simulink model "snb_b_ser2par"  (R2012b)
settings: Solver=FixedStepDiscrete  SolverMode=SingleTasking  StartTime=0.0  StopTime=10000  RelTol=1e-3
undefined symbols (not defined in the file): Down, pfb_coeff_gen_calc, Up, xlipgetpartsetting
libraries: xbsIndex_r4 x8784, casper_library_misc x9, casper_library_communications x8, casper_library_delays x1, xps_library x1
(part 19 of 57)

== system snb_b_ser2par/unpack_and_reorder/fifo1 ==
  note: We are done transmitting if
      | we have reached the end
      | of the data, or are in reset
  note: We start off in reset and hold
      | reset high till the end of the first
      | packet we receive
  note: we do not allow writes to the data buffer if we know
      | that we are going to discard the current packet
  note: The flag buffer stores the word count
      | and flag associated with each packet
      | received. This is used to extract the
      | correct number of words and tag
      | it appropriately on the way out
  note: a fifo overflow should never happen
      | as extra packets are discarded
      | and packets that are too large
      | are also discarded.
      | Kept as a a sanity check
  note: discard new packet
      | if packet count
      | indicates already
      | at max we can
      | store
  note: We have received a good packet if
      | 1. discard line is low for whole time
      | 2. eof is high
      | 3. rx word count is the expected
      | multiple
      | 4.  rx word count is less than the
      | maximum allowed
      | 5. not discarding current packet due
      | to packet limit reached
      | 6. en is high
  note: clear discard on
      | last word of packet
  note: count up on last item of packet,
      | count down as last word leaves,
      | leave as is if both
  note: change tlag
      | as last data
      |  word leaves
  rst : Inport
  din : Inport  Port=2
  eof : Inport  Port=3
  en : Inport  Port=4
  discard : Inport  Port=5
  flagi : Inport  Port=6
  tx : Inport  Port=7
  Constant : xbsIndex_r4/Constant  const=2^scale_factor_bits-1  gui_display_data_type=Fixed-point  arith_type=Unsigned  n_bits=scale_factor_bits  bin_pt=0  preci_type=Single  exp_width=8  frac_width=24  explicit_period=on  period=1  equ=P=C  opselect=C  inp2=PCIN>>17  opr=+  inp1=P  carry=CIN  dbl_ovrd=off  block_type=constant
  Constant1 : xbsIndex_r4/Constant  const=0  gui_display_data_type=Boolean  arith_type=Boolean  n_bits=scale_factor_bits  bin_pt=0  preci_type=Single  exp_width=8  frac_width=24  explicit_period=on  period=1  equ=P=C  opselect=C  inp2=PCIN>>17  opr=+  inp1=P  carry=CIN  dbl_ovrd=off  block_type=constant
  Delay{,1..5,7..14} (14 alike) : xbsIndex_r4/Delay  rst=off  infoeditControl=Selection of Reset will increase slice count due to use of real FFs and instead of SRLs  en=off  latency=1  dbl_ovrd=off  reg_retiming=on  block_type=delay
      settings: block_version=11.4
  Delay6 : xbsIndex_r4/Delay  rst=on  infoeditControl=Selection of Reset will increase slice count due to use of real FFs and instead of SRLs  en=on  latency=1  dbl_ovrd=off  reg_retiming=on  block_type=delay
  Gateway Out{,1..20} (21 alike) : xbsIndex_r4/Gateway Out  inherit_from_input=off  hdl_port=on  timing_constraint=None  locs_specified=off  LOCs={}  UseAsDAC=off  DACChannel='1'  block_type=gatewayout
  Inverter{1..6} (6 alike) : xbsIndex_r4/Inverter  en=off  latency=0  dbl_ovrd=off  block_type=inv
  Logical{,3,5,11} (4 alike) : xbsIndex_r4/Logical  logical_function=AND  inputs=2  en=off  latency=0  precision=Full  arith_type=Unsigned  n_bits=16  bin_pt=0  align_bp=on  dbl_ovrd=off  block_type=logical
      Logical11 settings: block_version=11.4
  Logical1 : xbsIndex_r4/Logical  logical_function=AND  inputs=3  en=off  latency=0  precision=Full  arith_type=Unsigned  n_bits=16  bin_pt=0  align_bp=on  dbl_ovrd=off  block_type=logical
  Logical2 : xbsIndex_r4/Logical  logical_function=AND  inputs=6  en=off  latency=1  precision=Full  arith_type=Unsigned  n_bits=16  bin_pt=0  align_bp=on  dbl_ovrd=off  block_type=logical
  Logical{4,7..9} (4 alike) : xbsIndex_r4/Logical  logical_function=OR  inputs=2  en=off  latency=0  precision=Full  arith_type=Unsigned  n_bits=16  bin_pt=0  align_bp=on  dbl_ovrd=off  block_type=logical
      Logical7 settings: block_version=11.4
      Logical8 settings: block_version=11.4
      Logical9 settings: block_version=11.4
  Logical6 : xbsIndex_r4/Logical  logical_function=XOR  inputs=2  en=off  latency=0  precision=Full  arith_type=Unsigned  n_bits=16  bin_pt=0  align_bp=on  dbl_ovrd=off  block_type=logical
      settings: block_version=11.4
  Relational : xbsIndex_r4/Relational  mode=a=b  en=off  latency=0  dbl_ovrd=off  block_type=relational
  Slice : xbsIndex_r4/Slice  nbits=input_word_count_bits - scale_factor_bits  boolean_output=off  mode=Upper Bit Location + Width  bit1=0  base1=MSB of Input  bit0=0  base0=LSB of Input  dbl_ovrd=off  block_type=slice
  Terminator : Terminator
  Terminator1 : Terminator
  concat1 : xbsIndex_r4/Concat  num_inputs=2  dbl_ovrd=off  block_type=concat
  data_buffer : Subsystem  mask{depth_bits=input_word_count_bits+n_bits_depth, scale_factor=2^scale_factor_bits, full_bits=1, n_bits_in=n_bits_din, bram_latency=bram_latency}
      mask prompts: depth_bits "depth (2^?)"; scale_factor "output width scale factor"; full_bits "number of bits in %full signal"; n_bits_in "word size (bits)"; bram_latency "BRAM latency"
  discard_reg : xbsIndex_r4/Register  init=0  rst=on  en=on  dbl_ovrd=off  block_type=register
  discarding : xbsIndex_r4/Delay  rst=on  infoeditControl=Selection of Reset will increase slice count due to use of real FFs and instead of SRLs  en=on  latency=1  dbl_ovrd=off  reg_retiming=on  block_type=delay
      settings: block_version=11.4
  edge_detect : Subsystem  AncestorBlock=casper_library_misc/edge_detect  mask(edge_detect){edge=Rising, polarity=Active High, x_in=[0 0.08 0.08 0.16 0.16 0.24 0.24 0.32 0.32 0.4], y_in=[-1 -1  1  1  1  1  1  1  1  1], x_out=[0.6 0.68 0.68 0.76 0.76 0.84 0.84 0.92 0.92 1], y_out=[-1 -1  1  1 -1 -1 -1 -1 -1 -1]}
      mask prompts: edge "Edge Type"; polarity "Output Polarity"; x_in "Input X Positions"; y_in "Input Y Positions"; x_out "Output X Positions"; y_out "Output Y Positions"
      mask help: Output is active for one-cycle after each edge of the specified type (i.e. rising, falling or both).
      mask init: same as snb_b_ser2par/edge_detect
      settings: AttributesFormatString=|
      | rising edges
      | active high
      mask Help: Output is active for one-cycle after each edge of the specified type (i.e. rising, falling, or both).  Latency is zero.
      mask TypeOptions edge: Rising | Falling | Both
      mask TypeOptions polarity: Active High | Active Low
      mask Display:
      | plot(x_in_num,0.5+y_in_num*0.2);
      | plot(x_out_num,0.5+y_out_num*0.2);
  edge_detect1 : Subsystem  AncestorBlock=casper_library_misc/edge_detect  mask(edge_detect){edge=Falling, polarity=Active High, x_in=[0 0.08 0.08 0.16 0.16 0.24 0.24 0.32 0.32 0.4], y_in=[-1 -1  1  1  1  1  1  1  1  1], x_out=[0.6 0.68 0.68 0.76 0.76 0.84 0.84 0.92 0.92 1], y_out=[-1 -1  1  1 -1 -1 -1 -1 -1 -1]}
      mask prompts: edge "Edge Type"; polarity "Output Polarity"; x_in "Input X Positions"; y_in "Input Y Positions"; x_out "Output X Positions"; y_out "Output Y Positions"
      mask help: Output is active for one-cycle after each edge of the specified type (i.e. rising, falling or both).
      mask init: same as snb_b_ser2par/edge_detect
      settings: AttributesFormatString=|
      | falling edges
      | active high
      mask Help: Output is active for one-cycle after each edge of the specified type (i.e. rising, falling, or both).  Latency is zero.
      mask TypeOptions edge: Rising | Falling | Both
      mask TypeOptions polarity: Active High | Active Low
      mask Display:
      | plot(x_in_num,0.5+y_in_num*0.2);
      | plot(x_out_num,0.5+y_out_num*0.2);
  edge_detect2 : Subsystem  AncestorBlock=casper_library_misc/edge_detect  mask(edge_detect){edge=Rising, polarity=Active High, x_in=[0 0.08 0.08 0.16 0.16 0.24 0.24 0.32 0.32 0.4], y_in=[-1 -1  1  1  1  1  1  1  1  1], x_out=[0.6 0.68 0.68 0.76 0.76 0.84 0.84 0.92 0.92 1], y_out=[-1 -1  1  1 -1 -1 -1 -1 -1 -1]}
      mask prompts: edge "Edge Type"; polarity "Output Polarity"; x_in "Input X Positions"; y_in "Input Y Positions"; x_out "Output X Positions"; y_out "Output Y Positions"
      mask help: Output is active for one-cycle after each edge of the specified type (i.e. rising, falling or both).
      mask init: same as snb_b_ser2par/edge_detect
      settings: AttributesFormatString=|
      | rising edges
      | active high
      mask Help: Output is active for one-cycle after each edge of the specified type (i.e. rising, falling, or both).  Latency is zero.
      mask TypeOptions edge: Rising | Falling | Both
      mask TypeOptions polarity: Active High | Active Low
      mask Display:
      | plot(x_in_num,0.5+y_in_num*0.2);
      | plot(x_out_num,0.5+y_out_num*0.2);
  flag : xbsIndex_r4/Slice  nbits=n_bits_flag  boolean_output=off  mode=Lower Bit Location + Width  bit1=0  base1=MSB of Input  bit0=0  base0=LSB of Input  dbl_ovrd=off  block_type=slice
  flag_buffer : xbsIndex_r4/Dual Port RAM  depth=2^n_bits_depth  initVector=zeros(1, 2^n_bits_depth)  distributed_mem=Distributed memory  init_a=0  init_b=0  rst_a=off  rst_b=off  en_a=off  en_b=off  latency=1  write_mode_A=Read After Write  write_mode_B=Read After Write  dbl_ovrd=off  optimize=Area  block_type=dpram
  input : Scope  NumInputPorts=9
      settings: YMin=0~0~-1~0~3.25836e+46~5e+45~0~0~-5  YMax=1.2e+22~1~1~1~3.60134e+46~1.2e+46~1~750~5  SaveName=ScopeData4
  logical1 : xbsIndex_r4/Relational  mode=a=b  en=off  latency=0  dbl_ovrd=off  block_type=relational
  logical2 : xbsIndex_r4/Relational  mode=a>b  en=off  latency=1  dbl_ovrd=off  block_type=relational
  logical3 : xbsIndex_r4/Relational  mode=a=b  en=off  latency=1  dbl_ovrd=off  block_type=relational
  lsbs_wc : xbsIndex_r4/Slice  nbits=scale_factor_bits  boolean_output=off  mode=Lower Bit Location + Width  bit1=0  base1=MSB of Input  bit0=0  base0=LSB of Input  dbl_ovrd=off  block_type=slice
  msb_wc : xbsIndex_r4/Slice  nbits=1  boolean_output=on  mode=Upper Bit Location + Width  bit1=0  base1=MSB of Input  bit0=0  base0=LSB of Input  dbl_ovrd=off  block_type=slice
  output : Scope  NumInputPorts=7
      settings: YMin=-1~-1~-1~-1~-1~-1~-5  YMax=1~1~1~1~1~1~5  SaveName=ScopeData5
  output1 : Scope  NumInputPorts=5
      settings: YMin=0~0~0~0~0  YMax=1~1~600~1~300  SaveName=ScopeData8
  packet_count : xbsIndex_r4/Counter  cnt_type=Free Running  cnt_to=Inf  operation=Up/Down  start_count=0  cnt_by_val=1  arith_type=Unsigned  n_bits=n_bits_depth  bin_pt=0  load_pin=off  rst=on  en=on  explicit_period=on  period=1  dbl_ovrd=off  use_behavioral_HDL=on  implementation=Fabric  block_type=counter
  rd_add : xbsIndex_r4/Counter  cnt_type=Free Running  cnt_to=Inf  operation=Up  start_count=0  cnt_by_val=1  arith_type=Unsigned  n_bits=n_bits_depth  bin_pt=0  load_pin=off  rst=on  en=on  explicit_period=on  period=1  dbl_ovrd=off  use_behavioral_HDL=on  implementation=Fabric  block_type=counter
      settings: block_version=11.4
  rst_reg : xbsIndex_r4/Register  init=1  rst=on  en=on  dbl_ovrd=off  block_type=register
  word_count : xbsIndex_r4/Slice  nbits=input_word_count_bits  boolean_output=off  mode=Upper Bit Location + Width  bit1=0  base1=MSB of Input  bit0=0  base0=LSB of Input  dbl_ovrd=off  block_type=slice
  word_count1 : xbsIndex_r4/Slice  nbits=input_word_count_bits  boolean_output=off  mode=Lower Bit Location + Width  bit1=0  base1=MSB of Input  bit0=0  base0=LSB of Input  dbl_ovrd=off  block_type=slice
  word_count_in : xbsIndex_r4/Counter  cnt_type=Free Running  cnt_to=inf  operation=Up  start_count=0  cnt_by_val=1  arith_type=Unsigned  n_bits=input_word_count_bits + 1  bin_pt=0  load_pin=off  rst=on  en=on  explicit_period=on  period=1  dbl_ovrd=off  use_behavioral_HDL=on  implementation=Fabric  block_type=counter
  word_count_out : xbsIndex_r4/Counter  cnt_type=Free Running  cnt_to=inf  operation=Up  start_count=0  cnt_by_val=1  arith_type=Unsigned  n_bits=input_word_count_bits - scale_factor_bits  bin_pt=0  load_pin=off  rst=on  en=on  explicit_period=on  period=1  dbl_ovrd=off  use_behavioral_HDL=on  implementation=Fabric  block_type=counter
  wr_addr : xbsIndex_r4/Counter  cnt_type=Free Running  cnt_to=Inf  operation=Up  start_count=0  cnt_by_val=1  arith_type=Unsigned  n_bits=n_bits_depth  bin_pt=0  load_pin=off  rst=on  en=on  explicit_period=on  period=1  dbl_ovrd=off  use_behavioral_HDL=on  implementation=Fabric  block_type=counter
      settings: block_version=11.4
  zero : xbsIndex_r4/Constant  const=0  gui_display_data_type=Fixed-point  arith_type=Unsigned  n_bits=n_bits_depth  bin_pt=0  preci_type=Single  exp_width=8  frac_width=24  explicit_period=on  period=1  equ=P=C  opselect=C  inp2=PCIN>>17  opr=+  inp1=P  carry=CIN  dbl_ovrd=off  block_type=constant
  zero1 : xbsIndex_r4/Constant  const=0  gui_display_data_type=Fixed-point  arith_type=Unsigned  n_bits=2  bin_pt=0  preci_type=Single  exp_width=8  frac_width=24  explicit_period=on  period=1  equ=P=C  opselect=C  inp2=PCIN>>17  opr=+  inp1=P  carry=CIN  dbl_ovrd=off  block_type=constant
  zero2 : xbsIndex_r4/Constant  const=0  gui_display_data_type=Fixed-point  arith_type=Unsigned  n_bits=2  bin_pt=0  preci_type=Single  exp_width=8  frac_width=24  explicit_period=on  period=1  equ=P=C  opselect=C  inp2=PCIN>>17  opr=+  inp1=P  carry=CIN  dbl_ovrd=off  block_type=constant
  zero3 : xbsIndex_r4/Constant  const=2^n_bits_depth-1  gui_display_data_type=Fixed-point  arith_type=Unsigned  n_bits=n_bits_depth  bin_pt=0  preci_type=Single  exp_width=8  frac_width=24  explicit_period=on  period=1  equ=P=C  opselect=C  inp2=PCIN>>17  opr=+  inp1=P  carry=CIN  dbl_ovrd=off  block_type=constant
  dout : Outport
  flago : Outport  Port=2
  dvalid : Outport  Port=3
  done : Outport  Port=4
  ready : Outport  Port=5
  fifo_of : Outport  Port=6
  discading : Outport  Port=7
  wires:
  Logical/1 -> Logical8/2, discard_reg/3, discard_reg/1
  [rst_in] -> rd_add/1
  data_buffer/4(dvalid) -> Delay4/1, edge_detect1/1(in)
  wr_addr/1 -> Gateway Out3/1, flag_buffer/1
  en/1 -> Logical2/6, Delay14/1, word_count_in/2, Logical3/2, Logical/1, Delay2/1
  [rst_in] -> data_buffer/1(rst_rx)
  din/1 -> Delay1/1
  [rst_in] -> wr_addr/1
  data_buffer/2(of) -> Delay5/1
  data_buffer/3(dout) -> Delay3/1
  Delay6/1 -> word_count_out/2, [tx]
  [tx] -> data_buffer/4(re)
  Delay1/1 -> data_buffer/3(din), Gateway Out/1
  [done] -> Delay6/2
  Delay3/1 -> dout/1
  Delay5/1 -> fifo_of/1
  [good_eof] -> wr_addr/2
  flagi/1 -> Delay/1
  concat1/1 -> flag_buffer/2
  [done] -> word_count_out/1
  Delay/1 -> concat1/2
  flag_buffer/2 -> flag/1, word_count/1
  flag/1 -> flago/1
  word_count/1 -> [input_count]
  [input_count] -> Slice/1
  word_count_out/1 -> logical1/1, Delay9/1, Gateway Out18/1
  Slice/1 -> logical1/2
  edge_detect1/1(out) -> done/1, rd_add/2
  data_buffer/1(%full) -> Terminator/1
  zero/1 -> logical2/2
  packet_count/1 -> logical2/1, Delay12/1, logical3/1
  [rst_in] -> packet_count/2
  edge_detect/1(out) -> Logical6/1
  Delay4/1 -> Gateway Out19/1, dvalid/1
  [rst_in] -> Logical7/1
  Logical7/1 -> discard_reg/2
  Logical8/1 -> Gateway Out2/1, Inverter2/1
  Logical6/1 -> Delay8/1, packet_count/3
  Gateway Out/1 -> input/1
  Gateway Out1/1 -> input/2
  Gateway Out2/1 -> input/3
  Gateway Out3/1 -> input/4
  Gateway Out4/1 -> input/5
  Gateway Out5/1 -> input/6
  Gateway Out6/1 -> input/7
  [ready] -> Gateway Out6/1
  [good_eof] -> Delay7/1
  [tx] -> Delay10/1
  Delay7/1 -> Gateway Out7/1
  Delay9/1 -> Gateway Out8/1
  Delay10/1 -> Gateway Out9/1
  Gateway Out10/1 -> input/8
  Delay11/1 -> [count_in], Gateway Out10/1, concat1/1
  Logical11/1 -> [done]
  Delay12/1 -> Gateway Out11/1
  [tx] -> Logical11/2
  tx/1 -> Delay6/1, Delay6/3
  logical2/1 -> Gateway Out12/1, ready/1, [ready]
  Delay13/1 -> [eof]
  [done] -> Gateway Out14/1
  Gateway Out14/1 -> output1/1
  [tx] -> Gateway Out15/1
  [input_count] -> Gateway Out16/1
  Gateway Out16/1 -> output1/3
  [done] -> Gateway Out13/1
  Gateway Out13/1 -> output1/4
  Gateway Out15/1 -> output1/2
  [tx] -> edge_detect/1(in)
  Delay2/1 -> Logical1/3, Gateway Out1/1
  eof/1 -> Delay13/1, Logical7/2, Logical2/2, Logical4/2, word_count_in/1
  Gateway Out17/1 -> output/6
  Gateway Out7/1 -> output/1
  Gateway Out9/1 -> output/3
  Gateway Out12/1 -> output/5
  Gateway Out11/1 -> output/4
  Gateway Out8/1 -> output/2
  word_count_in/1 -> msb_wc/1, lsbs_wc/1, word_count1/1
  Delay8/1 -> Gateway Out17/1
  [good_eof] -> packet_count/1
  Gateway Out18/1 -> output1/5
  [good_eof] -> Logical6/2
  Gateway Out19/1 -> output/7
  Delay14/1 -> flag_buffer/3
  Relational/1 -> Logical2/3
  Logical2/1 -> [good_eof]
  [eof] -> data_buffer/5(eof)
  [good_eof] -> Inverter3/1
  Gateway Out20/1 -> input/9
  [good_eof] -> Gateway Out20/1
  Logical5/1 -> edge_detect2/1(in), data_buffer/6(discard)
  Inverter3/1 -> Logical5/1
  [eof] -> Logical5/2
  rd_add/1 -> flag_buffer/4
  flag_buffer/1 -> Terminator1/1
  zero1/1 -> Gateway Out4/1
  zero2/1 -> Gateway Out5/1
  [pkt_max] -> Logical3/1
  Logical3/1 -> discarding/1, discarding/3
  discarding/1 -> Inverter1/1, [discarding]
  Constant/1 -> Relational/1
  lsbs_wc/1 -> Relational/2
  [word_max] -> Inverter4/1
  [rst_in] -> Logical4/1
  Logical4/1 -> discarding/2
  Inverter2/1 -> Logical2/1
  Inverter4/1 -> Logical2/4
  logical3/1 -> [pkt_max]
  Inverter1/1 -> Logical2/5
  discard/1 -> Logical/2
  discard_reg/1 -> Logical8/1
  Logical1/1 -> data_buffer/2(we)
  Inverter5/1 -> Logical1/2
  Inverter6/1 -> Logical1/1
  msb_wc/1 -> [word_max]
  [word_max] -> Inverter5/1
  [discarding] -> Inverter6/1
  edge_detect2/1(out) -> discading/1
  word_count1/1 -> Delay11/1
  zero3/1 -> logical3/2
  rst/1 -> rst_reg/2
  Constant1/1 -> rst_reg/1
  [eof] -> rst_reg/3
  rst_reg/1 -> [rst_in]
  logical1/1 -> Logical9/2
  Logical9/1 -> Logical11/1
  [rst_in] -> Logical9/1

== system snb_b_ser2par/unpack_and_reorder/fifo2 ==
  note: change tlag
      | as last data
      |  word leaves
  note: count up on last item of packet,
      | count down as last word leaves,
      | leave as is if both
  note: clear discard on
      | last word of packet
  note: We have received a good packet if
      | 1. discard line is low for whole time
      | 2. eof is high
      | 3. rx word count is the expected
      | multiple
      | 4.  rx word count is less than the
      | maximum allowed
      | 5. not discarding current packet due
      | to packet limit reached
      | 6. en is high
  note: discard new packet
      | if packet count
      | indicates already
      | at max we can
      | store
  note: a fifo overflow should never happen
      | as extra packets are discarded
      | and packets that are too large
      | are also discarded.
      | Kept as a a sanity check
  note: The flag buffer stores the word count
      | and flag associated with each packet
      | received. This is used to extract the
      | correct number of words and tag
      | it appropriately on the way out
  note: we do not allow writes to the data buffer if we know
      | that we are going to discard the current packet
  note: We start off in reset and hold
      | reset high till the end of the first
      | packet we receive
  note: We are done transmitting if
      | we have reached the end
      | of the data, or are in reset
  rst : Inport
  din : Inport  Port=2
  eof : Inport  Port=3
  en : Inport  Port=4
  discard : Inport  Port=5
  flagi : Inport  Port=6
  tx : Inport  Port=7
  Constant : xbsIndex_r4/Constant  const=2^scale_factor_bits-1  gui_display_data_type=Fixed-point  arith_type=Unsigned  n_bits=scale_factor_bits  bin_pt=0  preci_type=Single  exp_width=8  frac_width=24  explicit_period=on  period=1  equ=P=C  opselect=C  inp2=PCIN>>17  opr=+  inp1=P  carry=CIN  dbl_ovrd=off  block_type=constant
  Constant1 : xbsIndex_r4/Constant  const=0  gui_display_data_type=Boolean  arith_type=Boolean  n_bits=scale_factor_bits  bin_pt=0  preci_type=Single  exp_width=8  frac_width=24  explicit_period=on  period=1  equ=P=C  opselect=C  inp2=PCIN>>17  opr=+  inp1=P  carry=CIN  dbl_ovrd=off  block_type=constant
  Delay{,1..5,7..14} (14 alike) : xbsIndex_r4/Delay  rst=off  infoeditControl=Selection of Reset will increase slice count due to use of real FFs and instead of SRLs  en=off  latency=1  dbl_ovrd=off  reg_retiming=on  block_type=delay
      settings: block_version=11.4
  Delay6 : xbsIndex_r4/Delay  rst=on  infoeditControl=Selection of Reset will increase slice count due to use of real FFs and instead of SRLs  en=on  latency=1  dbl_ovrd=off  reg_retiming=on  block_type=delay
  Gateway Out{,1..20} (21 alike) : xbsIndex_r4/Gateway Out  inherit_from_input=off  hdl_port=on  timing_constraint=None  locs_specified=off  LOCs={}  UseAsDAC=off  DACChannel='1'  block_type=gatewayout
  Inverter{1..6} (6 alike) : xbsIndex_r4/Inverter  en=off  latency=0  dbl_ovrd=off  block_type=inv
  Logical{,3,5,11} (4 alike) : xbsIndex_r4/Logical  logical_function=AND  inputs=2  en=off  latency=0  precision=Full  arith_type=Unsigned  n_bits=16  bin_pt=0  align_bp=on  dbl_ovrd=off  block_type=logical
      Logical11 settings: block_version=11.4
  Logical1 : xbsIndex_r4/Logical  logical_function=AND  inputs=3  en=off  latency=0  precision=Full  arith_type=Unsigned  n_bits=16  bin_pt=0  align_bp=on  dbl_ovrd=off  block_type=logical
  Logical2 : xbsIndex_r4/Logical  logical_function=AND  inputs=6  en=off  latency=1  precision=Full  arith_type=Unsigned  n_bits=16  bin_pt=0  align_bp=on  dbl_ovrd=off  block_type=logical
  Logical{4,7..9} (4 alike) : xbsIndex_r4/Logical  logical_function=OR  inputs=2  en=off  latency=0  precision=Full  arith_type=Unsigned  n_bits=16  bin_pt=0  align_bp=on  dbl_ovrd=off  block_type=logical
      Logical7 settings: block_version=11.4
      Logical8 settings: block_version=11.4
      Logical9 settings: block_version=11.4
  Logical6 : xbsIndex_r4/Logical  logical_function=XOR  inputs=2  en=off  latency=0  precision=Full  arith_type=Unsigned  n_bits=16  bin_pt=0  align_bp=on  dbl_ovrd=off  block_type=logical
      settings: block_version=11.4
  Relational : xbsIndex_r4/Relational  mode=a=b  en=off  latency=0  dbl_ovrd=off  block_type=relational
  Slice : xbsIndex_r4/Slice  nbits=input_word_count_bits - scale_factor_bits  boolean_output=off  mode=Upper Bit Location + Width  bit1=0  base1=MSB of Input  bit0=0  base0=LSB of Input  dbl_ovrd=off  block_type=slice
  Terminator : Terminator
  Terminator1 : Terminator
  concat1 : xbsIndex_r4/Concat  num_inputs=2  dbl_ovrd=off  block_type=concat
  data_buffer : Subsystem  mask{depth_bits=input_word_count_bits+n_bits_depth, scale_factor=2^scale_factor_bits, full_bits=1, n_bits_in=n_bits_din, bram_latency=bram_latency}
      mask prompts: depth_bits "depth (2^?)"; scale_factor "output width scale factor"; full_bits "number of bits in %full signal"; n_bits_in "word size (bits)"; bram_latency "BRAM latency"
  discard_reg : xbsIndex_r4/Register  init=0  rst=on  en=on  dbl_ovrd=off  block_type=register
  discarding : xbsIndex_r4/Delay  rst=on  infoeditControl=Selection of Reset will increase slice count due to use of real FFs and instead of SRLs  en=on  latency=1  dbl_ovrd=off  reg_retiming=on  block_type=delay
      settings: block_version=11.4
  edge_detect : Subsystem  AncestorBlock=casper_library_misc/edge_detect  mask(edge_detect){edge=Rising, polarity=Active High, x_in=[0 0.08 0.08 0.16 0.16 0.24 0.24 0.32 0.32 0.4], y_in=[-1 -1  1  1  1  1  1  1  1  1], x_out=[0.6 0.68 0.68 0.76 0.76 0.84 0.84 0.92 0.92 1], y_out=[-1 -1  1  1 -1 -1 -1 -1 -1 -1]}
      mask prompts: edge "Edge Type"; polarity "Output Polarity"; x_in "Input X Positions"; y_in "Input Y Positions"; x_out "Output X Positions"; y_out "Output Y Positions"
      mask help: Output is active for one-cycle after each edge of the specified type (i.e. rising, falling or both).
      mask init: same as snb_b_ser2par/edge_detect
      settings: AttributesFormatString=|
      | rising edges
      | active high
      mask Help: Output is active for one-cycle after each edge of the specified type (i.e. rising, falling, or both).  Latency is zero.
      mask TypeOptions edge: Rising | Falling | Both
      mask TypeOptions polarity: Active High | Active Low
      mask Display:
      | plot(x_in_num,0.5+y_in_num*0.2);
      | plot(x_out_num,0.5+y_out_num*0.2);
  edge_detect1 : Subsystem  AncestorBlock=casper_library_misc/edge_detect  mask(edge_detect){edge=Falling, polarity=Active High, x_in=[0 0.08 0.08 0.16 0.16 0.24 0.24 0.32 0.32 0.4], y_in=[-1 -1  1  1  1  1  1  1  1  1], x_out=[0.6 0.68 0.68 0.76 0.76 0.84 0.84 0.92 0.92 1], y_out=[-1 -1  1  1 -1 -1 -1 -1 -1 -1]}
      mask prompts: edge "Edge Type"; polarity "Output Polarity"; x_in "Input X Positions"; y_in "Input Y Positions"; x_out "Output X Positions"; y_out "Output Y Positions"
      mask help: Output is active for one-cycle after each edge of the specified type (i.e. rising, falling or both).
      mask init: same as snb_b_ser2par/edge_detect
      settings: AttributesFormatString=|
      | falling edges
      | active high
      mask Help: Output is active for one-cycle after each edge of the specified type (i.e. rising, falling, or both).  Latency is zero.
      mask TypeOptions edge: Rising | Falling | Both
      mask TypeOptions polarity: Active High | Active Low
      mask Display:
      | plot(x_in_num,0.5+y_in_num*0.2);
      | plot(x_out_num,0.5+y_out_num*0.2);
  edge_detect2 : Subsystem  AncestorBlock=casper_library_misc/edge_detect  mask(edge_detect){edge=Rising, polarity=Active High, x_in=[0 0.08 0.08 0.16 0.16 0.24 0.24 0.32 0.32 0.4], y_in=[-1 -1  1  1  1  1  1  1  1  1], x_out=[0.6 0.68 0.68 0.76 0.76 0.84 0.84 0.92 0.92 1], y_out=[-1 -1  1  1 -1 -1 -1 -1 -1 -1]}
      mask prompts: edge "Edge Type"; polarity "Output Polarity"; x_in "Input X Positions"; y_in "Input Y Positions"; x_out "Output X Positions"; y_out "Output Y Positions"
      mask help: Output is active for one-cycle after each edge of the specified type (i.e. rising, falling or both).
      mask init: same as snb_b_ser2par/edge_detect
      settings: AttributesFormatString=|
      | rising edges
      | active high
      mask Help: Output is active for one-cycle after each edge of the specified type (i.e. rising, falling, or both).  Latency is zero.
      mask TypeOptions edge: Rising | Falling | Both
      mask TypeOptions polarity: Active High | Active Low
      mask Display:
      | plot(x_in_num,0.5+y_in_num*0.2);
      | plot(x_out_num,0.5+y_out_num*0.2);
  flag : xbsIndex_r4/Slice  nbits=n_bits_flag  boolean_output=off  mode=Lower Bit Location + Width  bit1=0  base1=MSB of Input  bit0=0  base0=LSB of Input  dbl_ovrd=off  block_type=slice
  flag_buffer : xbsIndex_r4/Dual Port RAM  depth=2^n_bits_depth  initVector=zeros(1, 2^n_bits_depth)  distributed_mem=Distributed memory  init_a=0  init_b=0  rst_a=off  rst_b=off  en_a=off  en_b=off  latency=1  write_mode_A=Read After Write  write_mode_B=Read After Write  dbl_ovrd=off  optimize=Area  block_type=dpram
  input : Scope  NumInputPorts=9
      settings: YMin=0~0~-1~0~3.25836e+46~5e+45~0~0~-5  YMax=1.2e+22~1~1~1~3.60134e+46~1.2e+46~1~750~5  SaveName=ScopeData4
  logical1 : xbsIndex_r4/Relational  mode=a=b  en=off  latency=0  dbl_ovrd=off  block_type=relational
  logical2 : xbsIndex_r4/Relational  mode=a>b  en=off  latency=1  dbl_ovrd=off  block_type=relational
  logical3 : xbsIndex_r4/Relational  mode=a=b  en=off  latency=1  dbl_ovrd=off  block_type=relational
  lsbs_wc : xbsIndex_r4/Slice  nbits=scale_factor_bits  boolean_output=off  mode=Lower Bit Location + Width  bit1=0  base1=MSB of Input  bit0=0  base0=LSB of Input  dbl_ovrd=off  block_type=slice
  msb_wc : xbsIndex_r4/Slice  nbits=1  boolean_output=on  mode=Upper Bit Location + Width  bit1=0  base1=MSB of Input  bit0=0  base0=LSB of Input  dbl_ovrd=off  block_type=slice
  output : Scope  NumInputPorts=7
      settings: YMin=-1~-1~-1~-1~-1~-1~-5  YMax=1~1~1~1~1~1~5  SaveName=ScopeData5
  output1 : Scope  NumInputPorts=5
      settings: YMin=0~0~0~0~0  YMax=1~1~600~1~300  SaveName=ScopeData8
  packet_count : xbsIndex_r4/Counter  cnt_type=Free Running  cnt_to=Inf  operation=Up/Down  start_count=0  cnt_by_val=1  arith_type=Unsigned  n_bits=n_bits_depth  bin_pt=0  load_pin=off  rst=on  en=on  explicit_period=on  period=1  dbl_ovrd=off  use_behavioral_HDL=on  implementation=Fabric  block_type=counter
  rd_add : xbsIndex_r4/Counter  cnt_type=Free Running  cnt_to=Inf  operation=Up  start_count=0  cnt_by_val=1  arith_type=Unsigned  n_bits=n_bits_depth  bin_pt=0  load_pin=off  rst=on  en=on  explicit_period=on  period=1  dbl_ovrd=off  use_behavioral_HDL=on  implementation=Fabric  block_type=counter
      settings: block_version=11.4
  rst_reg : xbsIndex_r4/Register  init=1  rst=on  en=on  dbl_ovrd=off  block_type=register
  word_count : xbsIndex_r4/Slice  nbits=input_word_count_bits  boolean_output=off  mode=Upper Bit Location + Width  bit1=0  base1=MSB of Input  bit0=0  base0=LSB of Input  dbl_ovrd=off  block_type=slice
  word_count1 : xbsIndex_r4/Slice  nbits=input_word_count_bits  boolean_output=off  mode=Lower Bit Location + Width  bit1=0  base1=MSB of Input  bit0=0  base0=LSB of Input  dbl_ovrd=off  block_type=slice
  word_count_in : xbsIndex_r4/Counter  cnt_type=Free Running  cnt_to=inf  operation=Up  start_count=0  cnt_by_val=1  arith_type=Unsigned  n_bits=input_word_count_bits + 1  bin_pt=0  load_pin=off  rst=on  en=on  explicit_period=on  period=1  dbl_ovrd=off  use_behavioral_HDL=on  implementation=Fabric  block_type=counter
  word_count_out : xbsIndex_r4/Counter  cnt_type=Free Running  cnt_to=inf  operation=Up  start_count=0  cnt_by_val=1  arith_type=Unsigned  n_bits=input_word_count_bits - scale_factor_bits  bin_pt=0  load_pin=off  rst=on  en=on  explicit_period=on  period=1  dbl_ovrd=off  use_behavioral_HDL=on  implementation=Fabric  block_type=counter
  wr_addr : xbsIndex_r4/Counter  cnt_type=Free Running  cnt_to=Inf  operation=Up  start_count=0  cnt_by_val=1  arith_type=Unsigned  n_bits=n_bits_depth  bin_pt=0  load_pin=off  rst=on  en=on  explicit_period=on  period=1  dbl_ovrd=off  use_behavioral_HDL=on  implementation=Fabric  block_type=counter
      settings: block_version=11.4
  zero : xbsIndex_r4/Constant  const=0  gui_display_data_type=Fixed-point  arith_type=Unsigned  n_bits=n_bits_depth  bin_pt=0  preci_type=Single  exp_width=8  frac_width=24  explicit_period=on  period=1  equ=P=C  opselect=C  inp2=PCIN>>17  opr=+  inp1=P  carry=CIN  dbl_ovrd=off  block_type=constant
  zero1 : xbsIndex_r4/Constant  const=0  gui_display_data_type=Fixed-point  arith_type=Unsigned  n_bits=2  bin_pt=0  preci_type=Single  exp_width=8  frac_width=24  explicit_period=on  period=1  equ=P=C  opselect=C  inp2=PCIN>>17  opr=+  inp1=P  carry=CIN  dbl_ovrd=off  block_type=constant
  zero2 : xbsIndex_r4/Constant  const=0  gui_display_data_type=Fixed-point  arith_type=Unsigned  n_bits=2  bin_pt=0  preci_type=Single  exp_width=8  frac_width=24  explicit_period=on  period=1  equ=P=C  opselect=C  inp2=PCIN>>17  opr=+  inp1=P  carry=CIN  dbl_ovrd=off  block_type=constant
  zero3 : xbsIndex_r4/Constant  const=2^n_bits_depth-1  gui_display_data_type=Fixed-point  arith_type=Unsigned  n_bits=n_bits_depth  bin_pt=0  preci_type=Single  exp_width=8  frac_width=24  explicit_period=on  period=1  equ=P=C  opselect=C  inp2=PCIN>>17  opr=+  inp1=P  carry=CIN  dbl_ovrd=off  block_type=constant
  dout : Outport
  flago : Outport  Port=2
  dvalid : Outport  Port=3
  done : Outport  Port=4
  ready : Outport  Port=5
  fifo_of : Outport  Port=6
  discading : Outport  Port=7
  wires:
  [rst_in] -> Logical9/1
  Logical9/1 -> Logical11/1
  logical1/1 -> Logical9/2
  rst_reg/1 -> [rst_in]
  [eof] -> rst_reg/3
  Constant1/1 -> rst_reg/1
  rst/1 -> rst_reg/2
  zero3/1 -> logical3/2
  word_count1/1 -> Delay11/1
  edge_detect2/1(out) -> discading/1
  [discarding] -> Inverter6/1
  [word_max] -> Inverter5/1
  msb_wc/1 -> [word_max]
  Inverter6/1 -> Logical1/1
  Inverter5/1 -> Logical1/2
  Logical1/1 -> data_buffer/2(we)
  discard_reg/1 -> Logical8/1
  discard/1 -> Logical/2
  Inverter1/1 -> Logical2/5
  logical3/1 -> [pkt_max]
  Inverter4/1 -> Logical2/4
  Inverter2/1 -> Logical2/1
  Logical4/1 -> discarding/2
  [rst_in] -> Logical4/1
  [word_max] -> Inverter4/1
  lsbs_wc/1 -> Relational/2
  Constant/1 -> Relational/1
  discarding/1 -> [discarding], Inverter1/1
  Logical3/1 -> discarding/3, discarding/1
  [pkt_max] -> Logical3/1
  zero2/1 -> Gateway Out5/1
  zero1/1 -> Gateway Out4/1
  flag_buffer/1 -> Terminator1/1
  rd_add/1 -> flag_buffer/4
  [eof] -> Logical5/2
  Inverter3/1 -> Logical5/1
  Logical5/1 -> data_buffer/6(discard), edge_detect2/1(in)
  [good_eof] -> Gateway Out20/1
  Gateway Out20/1 -> input/9
  [good_eof] -> Inverter3/1
  [eof] -> data_buffer/5(eof)
  Logical2/1 -> [good_eof]
  Relational/1 -> Logical2/3
  Delay14/1 -> flag_buffer/3
  Gateway Out19/1 -> output/7
  [good_eof] -> Logical6/2
  Gateway Out18/1 -> output1/5
  [good_eof] -> packet_count/1
  Delay8/1 -> Gateway Out17/1
  word_count_in/1 -> word_count1/1, lsbs_wc/1, msb_wc/1
  Gateway Out8/1 -> output/2
  Gateway Out11/1 -> output/4
  Gateway Out12/1 -> output/5
  Gateway Out9/1 -> output/3
  Gateway Out7/1 -> output/1
  Gateway Out17/1 -> output/6
  eof/1 -> word_count_in/1, Logical4/2, Logical2/2, Logical7/2, Delay13/1
  Delay2/1 -> Gateway Out1/1, Logical1/3
  [tx] -> edge_detect/1(in)
  Gateway Out15/1 -> output1/2
  Gateway Out13/1 -> output1/4
  [done] -> Gateway Out13/1
  Gateway Out16/1 -> output1/3
  [input_count] -> Gateway Out16/1
  [tx] -> Gateway Out15/1
  Gateway Out14/1 -> output1/1
  [done] -> Gateway Out14/1
  Delay13/1 -> [eof]
  logical2/1 -> [ready], ready/1, Gateway Out12/1
  tx/1 -> Delay6/3, Delay6/1
  [tx] -> Logical11/2
  Delay12/1 -> Gateway Out11/1
  Logical11/1 -> [done]
  Delay11/1 -> concat1/1, Gateway Out10/1, [count_in]
  Gateway Out10/1 -> input/8
  Delay10/1 -> Gateway Out9/1
  Delay9/1 -> Gateway Out8/1
  Delay7/1 -> Gateway Out7/1
  [tx] -> Delay10/1
  [good_eof] -> Delay7/1
  [ready] -> Gateway Out6/1
  Gateway Out6/1 -> input/7
  Gateway Out5/1 -> input/6
  Gateway Out4/1 -> input/5
  Gateway Out3/1 -> input/4
  Gateway Out2/1 -> input/3
  Gateway Out1/1 -> input/2
  Gateway Out/1 -> input/1
  Logical6/1 -> packet_count/3, Delay8/1
  Logical8/1 -> Inverter2/1, Gateway Out2/1
  Logical7/1 -> discard_reg/2
  [rst_in] -> Logical7/1
  Delay4/1 -> dvalid/1, Gateway Out19/1
  edge_detect/1(out) -> Logical6/1
  [rst_in] -> packet_count/2
  packet_count/1 -> logical3/1, Delay12/1, logical2/1
  zero/1 -> logical2/2
  data_buffer/1(%full) -> Terminator/1
  edge_detect1/1(out) -> rd_add/2, done/1
  Slice/1 -> logical1/2
  word_count_out/1 -> Gateway Out18/1, Delay9/1, logical1/1
  [input_count] -> Slice/1
  word_count/1 -> [input_count]
  flag/1 -> flago/1
  flag_buffer/2 -> word_count/1, flag/1
  Delay/1 -> concat1/2
  [done] -> word_count_out/1
  concat1/1 -> flag_buffer/2
  flagi/1 -> Delay/1
  [good_eof] -> wr_addr/2
  Delay5/1 -> fifo_of/1
  Delay3/1 -> dout/1
  [done] -> Delay6/2
  Delay1/1 -> Gateway Out/1, data_buffer/3(din)
  [tx] -> data_buffer/4(re)
  Delay6/1 -> [tx], word_count_out/2
  data_buffer/3(dout) -> Delay3/1
  data_buffer/2(of) -> Delay5/1
  [rst_in] -> wr_addr/1
  din/1 -> Delay1/1
  [rst_in] -> data_buffer/1(rst_rx)
  en/1 -> Delay2/1, Logical/1, Logical3/2, word_count_in/2, Delay14/1, Logical2/6
  wr_addr/1 -> flag_buffer/1, Gateway Out3/1
  data_buffer/4(dvalid) -> edge_detect1/1(in), Delay4/1
  [rst_in] -> rd_add/1
  Logical/1 -> discard_reg/1, discard_reg/3, Logical8/2
